simulink model "motorRPMTest"  (R2025a)
settings: Solver=FixedStepAuto  StartTime=0.0  StopTime=inf  RelTol=1e-3  EnableMultiTasking=on
model workspace (MAT data in the model file):
  encoderDt = 0.01
  k_motor = 0.076
values from neighbouring files (symbols this model uses):
  A = [0   1          0                0 ... (first row only)    [AugmentedLQRTest.m]    (also in simpend.m)
  B = [ 0 ... (first row only)    [AugmentedLQRTest.m]    (also in simpend.m = [0; I/delta;0;m*l/delta])
  C = [1 0 0 0;0 0 1 0]    [simpend.m]
undefined symbols (not defined in the file or in its folder): Discrete, dspblkCoreblockFVToolHelper, gcbh, Time
libraries: arduinolib x3, simulink x1, ctrlSharedLib x1, dspstat3 x1
settings Model: DataTypeOverride=Single  SimulationMode=external  SILPILModeSetting=veronly  ExtModeTrigDuration=2  Creator=Hudso  LastModifiedBy=Hudso
settings SolverCC: AutoInsertRateTranBlk=on
settings OptimizationCC: EnhancedBackFolding=on  PassReuseOutputArgsAs=Individual arguments  ZeroExternalMemoryAtStartup=off  ZeroInternalMemoryAtStartup=off  MaxStackSize=64  OptimizeBlockOrder=speed  DifferentSizesBufferReuse=on  OptimizationCustomize=off  EfficientTunableParamExpr=on
settings DebuggingCC: ParameterTunabilityLossMsg=error
settings HardwareCC: ProdBitPerInt=16.0  ProdBitPerPointer=16.0  ProdBitPerSizeT=16.0  ProdBitPerPtrDiffT=16.0  ProdLargestAtomicFloat=None  ProdWordSize=8.0  ProdHWDeviceType=Atmel->AVR  UseEmbeddedCoderFeatures=off
settings SFSimCC: MATLABDynamicMemAlloc=off
settings RTWCC: SystemTargetFile=ert.tlc  HardwareBoard=Arduino Uno  TemplateMakefile=ert_default_tmf  Toolchain=Arduino AVR  BuildConfiguration=Faster Runs  Description=Embedded Coder
settings CodeAppCC: ForceParamTrailComments=on  IgnoreCustomStorageClasses=off  OperatorAnnotations=on  SimulinkDataObjDesc=on  SFDataObjDesc=on  InsertBlockDesc=on
settings ERTTargetCC: ExtModeTransport=3.0  ExtModeAutomaticAllocSize=off  ExtModeStaticAllocSize=250.0  InlinedParameterPlacement=Hierarchical  SupportContinuousTime=on  SupportNonInlinedSFcns=on  SupportVariableSizeSignals=on

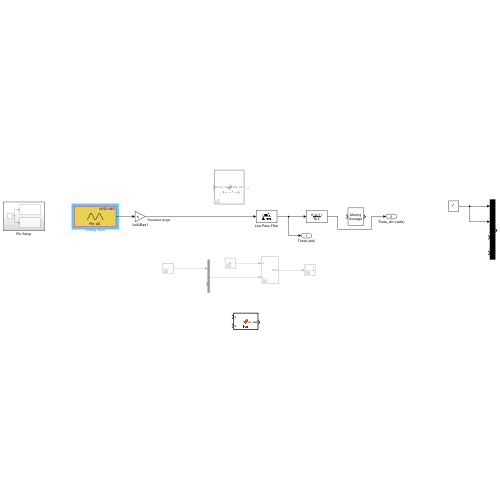
[thumbnail: Simulink's stored preview of the top-level diagram]
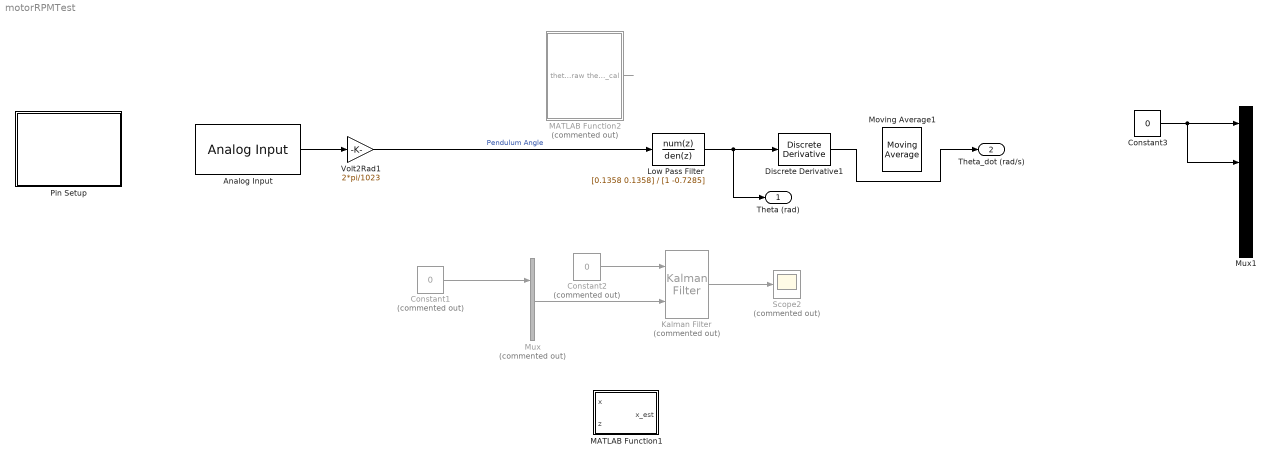
== system motorRPMTest ==
  Analog Input : arduinolib/Analog Input  pinNumber=0  ReadResultsOnly=off  ConversionTriggerSource=Software  ExternalTriggerType=uint32( 0 )  OutputDataType=uint16  EnableConversionCompleteNotify=off  EnableOuputStatus=off  SampleTime=0.01  blockPlatform=arduino
      settings: LibrarySourceBlock=gizmoLibrary/Arduino Utilities/Analog Input
  Constant1 : Constant  Commented=on  Value=0
  Constant2 : Constant  Commented=on  Value=0
  Constant3 : Constant  Value=0
  Discrete Derivative1 : simulink/Discrete/Discrete Derivative  gainval=1.0  ICPrevScaledInput=0.0  OutMin=[]  OutMax=[]  OutDataType=fixdt(1, 16)  OutScaling=2^-10  RndMeth=Nearest  DoSatur=off
  Kalman Filter : ctrlSharedLib/Kalman Filter  Commented=on  TimeDomain=Discrete-Time  UseCurrentEstimator=on  ModelSource=Individual A, B, C, D matrices  ModelSourceVariable=ss(0.95,1,1,0,1)  A=A  B=B  C=C  D=[0;0]  NumberOfStates=1  NumberOfInputs=1  NumberOfOutputs=1  InitialEstimateSource=Dialog  X0=0  P0=10  UseK=off  UseGH=off  NumberOfProcessNoiseInputs=1  G=1  TimeInvariantG=on  H=0  TimeInvariantH=on  Q=diag([0 0.01 0.01 0.03])  TimeInvariantQ=on  R=diag([0.01 .2])  TimeInvariantR=on  N=0  TimeInvariantN=on  AddInputPort=on  AddEnablePort=off  OutputEstimatedY=off  OutputP=off  Ts=-1
  Low Pass Filter : DiscreteTransferFcn  LoadFcn=dspblkCoreblockFVToolHelper(gcbh,'load');  Numerator=[0.1358 0.1358]  Denominator=[1 -0.7285]
      settings: CopyFcn=dspblkCoreblockFVToolHelper(gcbh,'copy');  DeleteFcn=dspblkCoreblockFVToolHelper(gcbh,'close');  ModelCloseFcn=dspblkCoreblockFVToolHelper(gcbh,'close');  PreSaveFcn=dspblkCoreblockFVToolHelper(gcbh,'presave');  PostSaveFcn=dspblkCoreblockFVToolHelper(gcbh,'postsave');  CloseFcn=dspblkCoreblockFVToolHelper(gcbh,'close');
  MATLAB Function1 : MATLAB Function  TreatAsAtomicUnit=on
  MATLAB Function2 : MATLAB Function  Commented=on  TreatAsAtomicUnit=on
  Moving Average1 : dspstat3/Moving Average  Method=Sliding window  ForgettingFactorPort=off  SpecifyWindowLength=on  WindowLength=2  OverlapLength=1  AllowArbitraryInputLength=off  ForgettingFactor=0.95  SimulateUsing=Interpreted execution
  Mux : Mux  Commented=on  Inputs=2
  Mux1 : Mux
  Pin Setup : Subsystem
  Scope2 : Scope  Commented=on
      settings: DataLoggingVariableName=ScopeData4
  Volt2Rad1 : Gain  Gain=2*pi/1023
  Theta (rad) : Outport
  Theta_dot (rad/s) : Outport  Port=2
  wires:
  Constant1/1 -> Mux/1
  Mux/1 -> Kalman Filter/2
  Kalman Filter/1 -> Scope2/1
  Constant2/1 -> Kalman Filter/1
  Constant3/1 -> Mux1/2, Mux1/1
  MATLAB Function2/1(theta_cal) -> ?
  Analog Input/1 -> Volt2Rad1/1
  Low Pass Filter/1 -> Discrete Derivative1/1, Theta (rad)/1
  Discrete Derivative1/1 -> Theta_dot (rad/s)/1
  Volt2Rad1/1 -> Low Pass Filter/1  "Pendulum Angle"

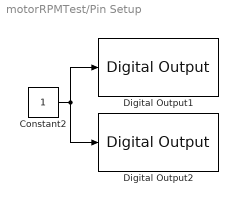
== system motorRPMTest/Pin Setup ==
  Constant2 : Constant
  Digital Output1 : arduinolib/Digital Output  pinNumber=7  Direction=output  blockPlatform=arduino
  Digital Output2 : arduinolib/Digital Output  pinNumber=8  Direction=output  blockPlatform=arduino
  wires:
  Constant2/1 -> Digital Output1/1, Digital Output2/1

== matlab function motorRPMTest/MATLAB Function2 ==
  data: theta_raw input; theta_cal output
function theta_cal = calibrateAngle(theta_raw)
% Calibrates angle by averaging first N samples at startup,
% then subtracting the average offset and adding pi.
%
% Inputs:
%  - theta_raw : current raw angle measurement
%  - reset     : boolean flag to reset calibration (true at startup)
%
% Output:
%  - theta_cal : calibrated angle (aligned so initial avg = pi)

    persistent sample_count theta_sum theta0 calibrated N

    if isempty(calibrated)
        % Initialization on reset
        N = 100;                % number of samples to average
        sample_count = 0;
        theta_sum = 0;
        theta0 = 0;
        calibrated = false;
    end

    if ~calibrated
        % Accumulate samples for averaging
        sample_count = sample_count + 1;
        theta_sum = theta_sum + theta_raw;
        
        if sample_count >= N
            theta0 = theta_sum / N;  % average offset
            calibrated = true;
        end
    end

    if calibrated
        % After calibration, subtract offset and add pi
        theta_cal = theta_raw - theta0 + 2*pi;
    else
        % During calibration phase, output raw angle
        theta_cal = theta_raw; 
    end
end

== matlab function motorRPMTest/MATLAB Function1 ==
  data: x input; x_est output; z input
function x_est = fcn(x, z)
% This function models a basic LKF for the pendulum system, linearized
% about the stable points. This does not output the covariance or residuals
% for simplicity of the calculation.
%
% Inputs:
% x = state vector (pos,vel,theta,theta_dot) [1x4]
% z = measurement (pos, theta)
%
% Outputs:
% y_est = state estimate

% --- Set up the Kalman Filter ---------------------------------------------

persistent Phi P R Q H

% These only needs to be calculated once, can store the value after. Check
% by seeing it Phi isempty to run this loop the first time
if isempty(Phi)

    % --- Model the Parameters of the Cart -------------------------------------

    m = 0.028; % mass of the pendulum arm (71 g for wood, 28g for CF)
    M = 0.408; % mass of the cart (408 g)
    l = 0.16; % length of pendulum arm (.16m for CF, 0.6096m for Wood)
    g = -9.81; % gravity
    I = (1/3) * m * l^2; % Moment of inertia for the pendulum

    % --- Build the state space ------------------------------------------------

    % define the denominator
    delta = I * (M+m) - (m*l)^2;

    % define the linearized control system
    A = [0   1          0                0;
        0   0   (m*l)^2*-g/delta        0;
        0   0          0                1;
        0   0   m*l*(M*-g+m*-g)/delta   0];

    %B = [0; I/delta;0;m*l/delta];

    H = [1 0 0 0;0 0 1 0];
    dt = 0.01;

    Phi = expm(A*dt);

    P = diag([0.005^2, ... % position uncertainty of 5 mm 1σ
        0.005^2, ... % velocity uncertainty of 5 mm/s 1σ
        0.01^2, ...  % angular uncertainty of 0.01 rad 1σ
        0.05^2]);    % angular vel. uncert. of 0.05 rad/s 1σ

    R = diag([0.001^2, 0.01^2]); % measurement uncertainty of 1 mm and 0.01 rad 1σ

    Q = diag([0.001^2, ... % position process noise of 1 mm 1σ
        0.001^2, ... % velocity process nosie of 1 mm/s 1σ
        0.005^2, ...  % angular process noise of 0.005 rad 1σ
        0.01^2]);    % angular vel. process noise of 0.01 rad/s 1σ
end


% --- Perform the Prediction Step ------------------------------------------

% get the current state (pos,vel,theta,theta_dot) and propagate it forward:
x_aPriori = Phi*x;

% Propagate the covariance:
P_aPriori = Phi*P*Phi' + Q;

% --- Perform the Measurement Update ---------------------------------------

% get the innovation:
y_est = z - H*x_aPriori;

% get the innovation
S = H*P_aPriori*H' + R;

% get the Kalman gain
K = P_aPriori*H' * inv(S);

% get the a posteriori state:
x_aPost = x_aPriori + K*y_est;

% get the a posteriori covariance
P_aPost = (eye(4)-K*H)*P_aPriori;

% save out variables for the next time step:
x_est = x_aPost;
P = P_aPost;
